simulink subsystem "PvtSubSys_VSM_LCK"  (R2020b)
settings: Solver=VariableStepAuto  StartTime=0.0  StopTime=10.0  RelTol=1e-3
values from neighbouring files (symbols this model uses):
  LCK_STATE : value not decoded    [LCK.sldd]
  P_VSM_LCK_A1 = 15.0    [LCK.sldd]
  P_VSM_LCK_AbsEspInTime = 3.0    [LCK.sldd]
  P_VSM_LCK_absLongitudeAccIn = 2.5    [LCK.sldd]
  P_VSM_LCK_absLongitudeAccOut = 3.0    [LCK.sldd]
  P_VSM_LCK_AccRateIn = 30.0    [LCK.sldd]
  P_VSM_LCK_AccRateInTime = 1.5    [LCK.sldd]
  P_VSM_LCK_AccRateOut = 80.0    [LCK.sldd]
  P_VSM_LCK_AccrPelOut = 30.0    [LCK.sldd]
  P_VSM_LCK_AccrPelRateOut = 0.0    [LCK.sldd]
  P_VSM_LCK_BrakePressIn = 3.0    [LCK.sldd]
  P_VSM_LCK_BrakePressInTime = 1.5    [LCK.sldd]
  P_VSM_LCK_BrakePressOut = 5.0    [LCK.sldd]
  P_VSM_LCK_C0 = 0.4    [LCK.sldd]
  P_VSM_LCK_DrvInputTrqValueIn = 2.0    [LCK.sldd]
  P_VSM_LCK_DrvInputTrqValueInTime = 3.0    [LCK.sldd]
  P_VSM_LCK_DrvInputTrqValueOut = 2.3    [LCK.sldd]
  P_VSM_LCK_dypreFactor = 1.0    [LCK.sldd]
  P_VSM_LCK_IdleInTime = 2.0    [LCK.sldd]
  P_VSM_LCK_LanechangeSwitch = 0.0    [LCK.sldd]
  P_VSM_LCK_LaneDouble = 1.0    [LCK.sldd]
  P_VSM_LCK_Lanewidthswitch = 1.0    [LCK.sldd]
  P_VSM_LCK_LateralAcceIn = 3.0    [LCK.sldd]
  P_VSM_LCK_LateralAcceInTime = 3.0    [LCK.sldd]
  P_VSM_LCK_LateralAcceOut = 3.5    [LCK.sldd]
  P_VSM_LCK_LCDrvInputTrqValueOut = 3.0    [LCK.sldd]
  P_VSM_LCK_LCOverrideTime = 0.6    [LCK.sldd]
  P_VSM_LCK_LCOverrideValue = 1.5    [LCK.sldd]
  P_VSM_LCK_LongitudeAccIn = 3.0    [LCK.sldd]
  P_VSM_LCK_LongitudeAccInTime = 3.0    [LCK.sldd]
  P_VSM_LCK_LongitudeAccOut = 3.5    [LCK.sldd]
  P_VSM_LCK_OverrideInTime = 3.0    [LCK.sldd]
  P_VSM_LCK_OverrideTime = 0.3    [LCK.sldd]
  P_VSM_LCK_OverrideValue = 1.2    [LCK.sldd]
  P_VSM_LCK_ParamA1 : value not decoded    [LCK.sldd]
  P_VSM_LCK_PreTime = 0.2    [LCK.sldd]
  P_VSM_LCK_State_Absesp_enable = 1.0    [LCK.sldd]
  P_VSM_LCK_State_Accpedalrate_enable = 0.0    [LCK.sldd]
  P_VSM_LCK_State_Breakpressure_enable = 1.0    [LCK.sldd]
  P_VSM_LCK_State_DriverInputTrqValue_enable = 1.0    [LCK.sldd]
  P_VSM_LCK_State_Eps_enable = 1.0    [LCK.sldd]
  P_VSM_LCK_State_ESSSts_enable = 1.0    [LCK.sldd]
  P_VSM_LCK_State_GEAR_enable = 1.0    [LCK.sldd]
  P_VSM_LCK_State_Handson_enable = 1.0    [LCK.sldd]
  P_VSM_LCK_State_IdleInTime_enable = 0.0    [LCK.sldd]
  P_VSM_LCK_State_Lane_enable = 1.0    [LCK.sldd]
  P_VSM_LCK_State_LaneChange_enable = 1.0    [LCK.sldd]
  P_VSM_LCK_State_LaneCurve_enable = 0.0    [LCK.sldd]
  P_VSM_LCK_State_LateralAcce_enable = 1.0    [LCK.sldd]
  P_VSM_LCK_State_LongitudeAcc_enable = 1.0    [LCK.sldd]
  P_VSM_LCK_State_LSMLine_enable = 1.0    [LCK.sldd]
  P_VSM_LCK_State_Overide_enable = 1.0    [LCK.sldd]
  P_VSM_LCK_State_Param_LaneCurve : value not decoded    [LCK.sldd]
  P_VSM_LCK_State_Param_LaneCurve_Offset : value not decoded    [LCK.sldd]
  P_VSM_LCK_State_Param_LaneWidth : value not decoded    [LCK.sldd]
  P_VSM_LCK_State_Param_LaneWidth_Offset : value not decoded    [LCK.sldd]
  P_VSM_LCK_State_SteerWheelAngle_enable = 1.0    [LCK.sldd]
  P_VSM_LCK_State_SteerWheelSpd_enable = 1.0    [LCK.sldd]
  P_VSM_LCK_State_TargetLaneIn_enable = 1.0    [LCK.sldd]
  P_VSM_LCK_State_TurnLight_enable = 1.0    [LCK.sldd]
  P_VSM_LCK_State_Vehspeed_enable = 1.0    [LCK.sldd]
  P_VSM_LCK_State_Yawsup_enable = 1.0    [LCK.sldd]
  P_VSM_LCK_SteerAngleSpdIn = 150.0    [LCK.sldd]
  P_VSM_LCK_SteerAngleSpdInTime = 3.0    [LCK.sldd]
  P_VSM_LCK_SteerAngleSpdOut = 200.0    [LCK.sldd]
  P_VSM_LCK_SteerWheelAngleIn = 70.0    [LCK.sldd]
  P_VSM_LCK_SteerWheelAngleInTime = 3.0    [LCK.sldd]
  P_VSM_LCK_SteerWheelAngleOut = 90.0    [LCK.sldd]
  P_VSM_LCK_T0 = 0.75    [LCK.sldd]
  P_VSM_LCK_T1 = 15.0    [LCK.sldd]
  P_VSM_LCK_TargetInSwitch = 0.0    [LCK.sldd]
  P_VSM_LCK_Warnarea1 = -0.55    [LCK.sldd]
  P_VSM_LCK_Warnarea2 = -0.35    [LCK.sldd]
  P_VSM_LCK_YawRateIn = 0.2    [LCK.sldd]
  P_VSM_LCK_YawRateInTime = 1.0    [LCK.sldd]
  P_VSM_LCK_YawRateOut = 0.25    [LCK.sldd]
undefined symbols (not defined in the file or in its folder): P_VSM_LSMC_SampleTime
libraries: simulink x275
(part 5 of 5)

== stateflow chart PvtSubSys_VSM_LCK/LCK2/LCK_StateMachine3/LCK_State ==
  state MAINST_ERROR
    en:State=LCK_STATE.LCK_Error;
  state MAINST_ON
    state SUBST_IDLE
      en: State=LCK_STATE.LCK_Idle;
    state enabled
      state SUBST_READY
        en:State=LCK_STATE.LCK_Ready;
      state SUBST_ACTIVE
        en:State=LCK_STATE.LCK_Active;
      (default) -> (junction 367)
      (junction 367) -> SUBST_READY [order 2]
      (junction 367) -> SUBST_ACTIVE [order 1] : [READY2ACTIVE]
      SUBST_READY -> SUBST_ACTIVE : [READY2ACTIVE]
      SUBST_ACTIVE -> SUBST_READY : [ACTIVE2READY]
    (junction 366) -> SUBST_IDLE [order 2]
    SUBST_IDLE -> enabled : [IDLE2READY]
    enabled -> SUBST_IDLE : [READY2IDLE]
    (default) -> (junction 366)
    (junction 366) -> enabled [order 1] : [IDLE2READY]
  MAINST_ON -> MAINST_ERROR : [LCKFailSts==1]
  MAINST_ERROR -> MAINST_ON : [LCKFailSts==0]
  (default) -> MAINST_ON
  data: LCKFailSts input; State output Enum: LCK_STATE =LCK_STATE.LCK_Off;; IDLE2READY input; READY2ACTIVE input; READY2IDLE input; ACTIVE2READY input

== matlab function PvtSubSys_VSM_LCK/LCK2/LCK_Condition1/Enlong3s3/MATLAB Function ==
  data: CntK1 input uint16; Cnt output uint16; X input; Num input
function Cnt= TextCount(CntK1,X,Num)

if X==true
    Cnt = Num;
else
     Cnt = max(CntK1-uint16(1),uint16(0));
end

== matlab function PvtSubSys_VSM_LCK/LCK2/LCK_Condition1/Enlong3s1/MATLAB Function ==
  data: CntK1 input uint16; Cnt output uint16; X input; Num input
function Cnt= TextCount(CntK1,X,Num)

if X==true
    Cnt = Num;
else
     Cnt = max(CntK1-uint16(1),uint16(0));
end

== matlab function PvtSubSys_VSM_LCK/LCK2/LCK/MATLAB Function ==
  data: preDis input; dy_pre output; kap input
function dy_pre = fcn(preDis, kap)
dy_pre = 0.5*kap*preDis^2;

== matlab function PvtSubSys_VSM_LCK/LCK2/LCK_Condition1/MATLAB Function1 ==
  data: HandsOff_Ready2Idle input; HandsOff_Ready2IdleK1 input; y output; LCKSts input; yK1 input
function y = fcn(HandsOff_Ready2Idle,HandsOff_Ready2IdleK1,LCKSts,yK1)
y=0;
if LCKSts==LCK_STATE.LCK_Idle
    if HandsOff_Ready2Idle==1 || HandsOff_Ready2IdleK1==1
        y=1;
    else
        y=yK1;
    end
elseif LCKSts~=LCK_STATE.LCK_Idle
    y=0;
end

== matlab function PvtSubSys_VSM_LCK/LCK2/LCK/MATLAB Function1 ==
  data: tCycle input; Vego input; A3 output; Kap input; LaneValid input; a3 input; a2 input; a1 input; a0 input; A2 output; A1 output; A0 output
function [A3,A2,A1,A0] = ...
    lckcenter(tCycle,Vego,Kap,LaneValid,a3,a2,a1,a0)

if Kap==single(0)
    dDeltaX = Vego*tCycle;
    dDeltaY = single(0);
    CosOfPsi = single(1);
    SinOfPsi = single(0);
else
    t_Psi = Kap*Vego*tCycle;
    SinOfPsi = sin(t_Psi);
    CosOfPsi = cos(t_Psi);
    dDeltaX = SinOfPsi/Kap;
    dDeltaY = 2*(sin(t_Psi/2)*sin(t_Psi/2))/Kap;
end

if (LaneValid)
t_Dist = max(single(15),Vego*1.8);
xi = [0.05*t_Dist;0.3*t_Dist;0.6*t_Dist;t_Dist];
yi = a3*xi.^3 + a2*xi.^2 + a1*xi + a0;
t_dx = xi-dDeltaX;
t_dy = yi-dDeltaY;
TmpX = t_dx*CosOfPsi+t_dy*SinOfPsi;
TmpY = -t_dx*SinOfPsi+t_dy*CosOfPsi;
[t3,t2,t1,t0] = pl(TmpX,TmpY);
A3 = t3;
A2 = t2;
A1 = t1;
A0 = t0;

else
A3 = single(0);
A2 = single(0);
A1 = single(0);
A0 = single(0);
end
    
end

== matlab function PvtSubSys_VSM_LCK/LCK2/LCK/MATLAB Function6 ==
  data: T_A2 input; Offset output; LaneCurveOffset input
function Offset = fcn(T_A2,LaneCurveOffset)
if T_A2==0
   Offset=0;
elseif T_A2>0
    Offset=LaneCurveOffset;
else
    Offset=-LaneCurveOffset;
end

== matlab function PvtSubSys_VSM_LCK/LCK2/LCK/MATLAB Function4 ==
  data: predis input; offset output; kap input; Dx input
function offset = fcn(predis,kap,Dx)
a=atan(kap*predis);
if kap==0
    offset=single(0);
else
    offset=Dx*sin(a);
end

== matlab function PvtSubSys_VSM_LCK/LCK2/LCK/MATLAB Function5 ==
  data: A0 input; dy0 output; A1 input; A2 input; A3 input; predis input
function dy0 = fcn(A0,A1,A2,A3,predis)
dy0=A0+A1*predis+A2*predis*predis+A3*predis*predis*predis;
